simulink subsystem "ALU_64bit_v2_SS"  (R2022a)
settings: Solver=VariableStepAuto  StartTime=0.0  StopTime=10.0  RelTol=1e-3
libraries: hdlBasic x192
(part 3 of 3)

== system ALU_64bit_v2_SS/alu 16bit3/Subsystem2 ==
  a : Inport
  b : Inport  Port=2
  Op : Inport  Port=3
  Ainv : Inport  Port=4
  Binv : Inport  Port=5
  CarryIn : Inport  Port=6
  Concat : hdlBasic/Concat  num_inputs=4  XmcBlockStatus=1  maskContainerNames=group1  block_type=concat  block_config=sysgen:Concat_config
  Slice : hdlBasic/Slice  nbits=1  boolean_output=off  mode=Upper Bit Location + Width  bit1=0  base1=LSB of Input  bit0=0  base0=LSB of Input  XmcBlockStatus=1  maskContainerNames=group1  block_type=slice  block_config=sysgen:Slice_config
  Slice1 : hdlBasic/Slice  nbits=1  boolean_output=off  mode=Upper Bit Location + Width  bit1=0  base1=LSB of Input  bit0=0  base0=LSB of Input  XmcBlockStatus=1  maskContainerNames=group1  block_type=slice  block_config=sysgen:Slice_config
  Slice2 : hdlBasic/Slice  nbits=1  boolean_output=off  mode=Upper Bit Location + Width  bit1=1  base1=LSB of Input  bit0=0  base0=LSB of Input  XmcBlockStatus=1  maskContainerNames=group1  block_type=slice  block_config=sysgen:Slice_config
  Slice3 : hdlBasic/Slice  nbits=1  boolean_output=off  mode=Upper Bit Location + Width  bit1=1  base1=LSB of Input  bit0=0  base0=LSB of Input  XmcBlockStatus=1  maskContainerNames=group1  block_type=slice  block_config=sysgen:Slice_config
  Slice4 : hdlBasic/Slice  nbits=1  boolean_output=off  mode=Upper Bit Location + Width  bit1=2  base1=LSB of Input  bit0=0  base0=LSB of Input  XmcBlockStatus=1  maskContainerNames=group1  block_type=slice  block_config=sysgen:Slice_config
  Slice5 : hdlBasic/Slice  nbits=1  boolean_output=off  mode=Upper Bit Location + Width  bit1=2  base1=LSB of Input  bit0=0  base0=LSB of Input  XmcBlockStatus=1  maskContainerNames=group1  block_type=slice  block_config=sysgen:Slice_config
  Slice6 : hdlBasic/Slice  nbits=1  boolean_output=off  mode=Upper Bit Location + Width  bit1=3  base1=LSB of Input  bit0=0  base0=LSB of Input  XmcBlockStatus=1  maskContainerNames=group1  block_type=slice  block_config=sysgen:Slice_config
  Slice7 : hdlBasic/Slice  nbits=1  boolean_output=off  mode=Upper Bit Location + Width  bit1=3  base1=LSB of Input  bit0=0  base0=LSB of Input  XmcBlockStatus=1  maskContainerNames=group1  block_type=slice  block_config=sysgen:Slice_config
  Subsystem Reference{,1..3} (4 alike) : Subsystem  ReferencedSubsystem=ALU_1bit_SS
      settings: PortSchema="{\"entries\":[{\"content\":{\"sides\":[{\"content\":{\"connectorIds\":[\"In4\",\"In5\"]},\"type\":\"ConnectorPlacement.EquallySpacedRectSide\",\"uuid\":\"2d8c2f3b-1550-46fa-bff2-1c6af3b5a107\"},{\"content\":{\"connectorIds\":[\"Out1\",\"Out2\"],\"side\":\"RIGHT\"},\"type\":\"ConnectorPlacement.EquallySpacedRectSide\",\"uuid\":\"4b8f41aa-218a-4e29-bd3a-77a8547f4b37\"},{\"content\":{\"connectorIds\":[\"In1\",\"In3\",\"In2\",\"In6\"],\"side\":\"TOP\"},\"type\":\"ConnectorPlacement.EquallySpacedRectSide\",\"uuid\":\"e119eb8d-dd79-436a-880b-8e6ed91d7b6a\"}]},\"type\":\"ConnectorPlacement.EquallySpacedConnector\",\"uuid\":\"6756e4eb-c638-4708-925d-61f35342c635\"}],\"packageUris\":[\"http://schema.mathworks.com/mf0/Connector/R2020b\"],\"version\":\"1.0\"}"
  result : Outport
  CarryOut : Outport  Port=2
  wires:
  Subsystem Reference3/1 -> Concat/1
  Subsystem Reference1/1 -> Concat/3
  Op/1 -> Subsystem Reference1/1, Subsystem Reference2/1, Subsystem Reference3/1, Subsystem Reference/1
  a/1 -> Slice/1, Slice2/1, Slice4/1, Slice6/1
  CarryIn/1 -> Subsystem Reference/6
  Binv/1 -> Subsystem Reference1/3, Subsystem Reference2/3, Subsystem Reference3/3, Subsystem Reference/3
  Ainv/1 -> Subsystem Reference1/2, Subsystem Reference2/2, Subsystem Reference3/2, Subsystem Reference/2
  Concat/1 -> result/1
  Slice4/1 -> Subsystem Reference2/4
  Subsystem Reference2/1 -> Concat/2
  Subsystem Reference1/2 -> Subsystem Reference2/6
  Slice6/1 -> Subsystem Reference3/4
  Slice7/1 -> Subsystem Reference3/5
  Slice5/1 -> Subsystem Reference2/5
  b/1 -> Slice1/1, Slice3/1, Slice5/1, Slice7/1
  Subsystem Reference/2 -> Subsystem Reference1/6
  Subsystem Reference2/2 -> Subsystem Reference3/6
  Subsystem Reference/1 -> Concat/4
  Slice/1 -> Subsystem Reference/4
  Subsystem Reference3/2 -> CarryOut/1
  Slice3/1 -> Subsystem Reference1/5
  Slice1/1 -> Subsystem Reference/5
  Slice2/1 -> Subsystem Reference1/4

== system ALU_64bit_v2_SS/alu 16bit3/Subsystem3 ==
  a : Inport
  b : Inport  Port=2
  Op : Inport  Port=3
  Ainv : Inport  Port=4
  Binv : Inport  Port=5
  CarryIn : Inport  Port=6
  Concat : hdlBasic/Concat  num_inputs=4  XmcBlockStatus=1  maskContainerNames=group1  block_type=concat  block_config=sysgen:Concat_config
  Slice : hdlBasic/Slice  nbits=1  boolean_output=off  mode=Upper Bit Location + Width  bit1=0  base1=LSB of Input  bit0=0  base0=LSB of Input  XmcBlockStatus=1  maskContainerNames=group1  block_type=slice  block_config=sysgen:Slice_config
  Slice1 : hdlBasic/Slice  nbits=1  boolean_output=off  mode=Upper Bit Location + Width  bit1=0  base1=LSB of Input  bit0=0  base0=LSB of Input  XmcBlockStatus=1  maskContainerNames=group1  block_type=slice  block_config=sysgen:Slice_config
  Slice2 : hdlBasic/Slice  nbits=1  boolean_output=off  mode=Upper Bit Location + Width  bit1=1  base1=LSB of Input  bit0=0  base0=LSB of Input  XmcBlockStatus=1  maskContainerNames=group1  block_type=slice  block_config=sysgen:Slice_config
  Slice3 : hdlBasic/Slice  nbits=1  boolean_output=off  mode=Upper Bit Location + Width  bit1=1  base1=LSB of Input  bit0=0  base0=LSB of Input  XmcBlockStatus=1  maskContainerNames=group1  block_type=slice  block_config=sysgen:Slice_config
  Slice4 : hdlBasic/Slice  nbits=1  boolean_output=off  mode=Upper Bit Location + Width  bit1=2  base1=LSB of Input  bit0=0  base0=LSB of Input  XmcBlockStatus=1  maskContainerNames=group1  block_type=slice  block_config=sysgen:Slice_config
  Slice5 : hdlBasic/Slice  nbits=1  boolean_output=off  mode=Upper Bit Location + Width  bit1=2  base1=LSB of Input  bit0=0  base0=LSB of Input  XmcBlockStatus=1  maskContainerNames=group1  block_type=slice  block_config=sysgen:Slice_config
  Slice6 : hdlBasic/Slice  nbits=1  boolean_output=off  mode=Upper Bit Location + Width  bit1=3  base1=LSB of Input  bit0=0  base0=LSB of Input  XmcBlockStatus=1  maskContainerNames=group1  block_type=slice  block_config=sysgen:Slice_config
  Slice7 : hdlBasic/Slice  nbits=1  boolean_output=off  mode=Upper Bit Location + Width  bit1=3  base1=LSB of Input  bit0=0  base0=LSB of Input  XmcBlockStatus=1  maskContainerNames=group1  block_type=slice  block_config=sysgen:Slice_config
  Subsystem Reference{,1..3} (4 alike) : Subsystem  ReferencedSubsystem=ALU_1bit_SS
      settings: PortSchema="{\"entries\":[{\"content\":{\"sides\":[{\"content\":{\"connectorIds\":[\"In4\",\"In5\"]},\"type\":\"ConnectorPlacement.EquallySpacedRectSide\",\"uuid\":\"2d8c2f3b-1550-46fa-bff2-1c6af3b5a107\"},{\"content\":{\"connectorIds\":[\"Out1\",\"Out2\"],\"side\":\"RIGHT\"},\"type\":\"ConnectorPlacement.EquallySpacedRectSide\",\"uuid\":\"4b8f41aa-218a-4e29-bd3a-77a8547f4b37\"},{\"content\":{\"connectorIds\":[\"In1\",\"In3\",\"In2\",\"In6\"],\"side\":\"TOP\"},\"type\":\"ConnectorPlacement.EquallySpacedRectSide\",\"uuid\":\"e119eb8d-dd79-436a-880b-8e6ed91d7b6a\"}]},\"type\":\"ConnectorPlacement.EquallySpacedConnector\",\"uuid\":\"6756e4eb-c638-4708-925d-61f35342c635\"}],\"packageUris\":[\"http://schema.mathworks.com/mf0/Connector/R2020b\"],\"version\":\"1.0\"}"
  result : Outport
  CarryOut : Outport  Port=2
  wires:
  Subsystem Reference3/1 -> Concat/1
  Subsystem Reference1/1 -> Concat/3
  Op/1 -> Subsystem Reference1/1, Subsystem Reference2/1, Subsystem Reference3/1, Subsystem Reference/1
  a/1 -> Slice/1, Slice2/1, Slice4/1, Slice6/1
  CarryIn/1 -> Subsystem Reference/6
  Binv/1 -> Subsystem Reference1/3, Subsystem Reference2/3, Subsystem Reference3/3, Subsystem Reference/3
  Ainv/1 -> Subsystem Reference1/2, Subsystem Reference2/2, Subsystem Reference3/2, Subsystem Reference/2
  Concat/1 -> result/1
  Slice4/1 -> Subsystem Reference2/4
  Subsystem Reference2/1 -> Concat/2
  Subsystem Reference1/2 -> Subsystem Reference2/6
  Slice6/1 -> Subsystem Reference3/4
  Slice7/1 -> Subsystem Reference3/5
  Slice5/1 -> Subsystem Reference2/5
  b/1 -> Slice1/1, Slice3/1, Slice5/1, Slice7/1
  Subsystem Reference/2 -> Subsystem Reference1/6
  Subsystem Reference2/2 -> Subsystem Reference3/6
  Subsystem Reference/1 -> Concat/4
  Slice/1 -> Subsystem Reference/4
  Subsystem Reference3/2 -> CarryOut/1
  Slice3/1 -> Subsystem Reference1/5
  Slice1/1 -> Subsystem Reference/5
  Slice2/1 -> Subsystem Reference1/4
